simulink subsystem "untimed_ctrl"  (R2021b)
settings: Solver=VariableStepAuto  StartTime=0.0  StopTime=10.0  RelTol=1e-3
undefined symbols (not defined in the file or in its folder): ls_bitwidth
settings Model: Creator=torha  LastModifiedBy=torha
settings SolverCC: AlgebraicLoopSolver=TrustRegion
settings DebuggingCC: SFMachineParentedDataDiag=warning

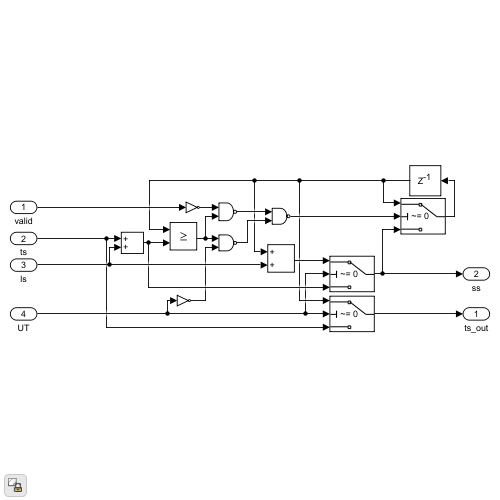
[thumbnail: Simulink's stored preview of the top-level diagram]
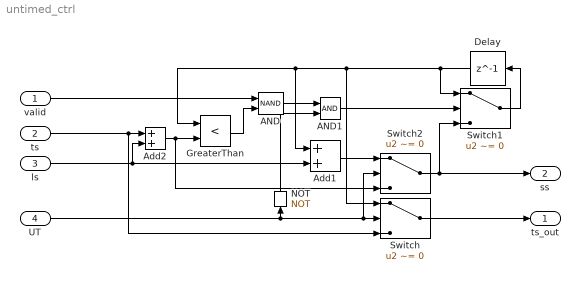
== system untimed_ctrl ==
  valid : Inport
  ts : Inport  Port=2
  ls : Inport  Port=3
  UT : Inport  Port=4
  AND : Logic  Operator=NAND  IconShape=distinctive  AllPortsSameDT=off  OutDataTypeStr=boolean
  AND1 : Logic  IconShape=distinctive  AllPortsSameDT=off  OutDataTypeStr=boolean
  Add1 : Sum  AccumDataTypeStr=fixdt(0,ls_bitwidth,0)
  Add2 : Sum  AccumDataTypeStr=fixdt(0,ls_bitwidth,0)
  Delay : Delay  DelayLength=1  InitialCondition=fi(0,0,ls_bitwidth,0)
  GreaterThan : RelationalOperator  Operator=<  OutDataTypeStr=boolean  RndMeth=Simplest
  NOT : Logic  Operator=NOT  IconShape=distinctive  AllPortsSameDT=off  OutDataTypeStr=boolean
  Switch : Switch  Criteria=u2 ~= 0
  Switch1 : Switch  Criteria=u2 ~= 0
  Switch2 : Switch  Criteria=u2 ~= 0
  ts_out : Outport
  ss : Outport  Port=2
  wires:
  ls/1 -> Add1/2, Add2/2
  Add1/1 -> Switch2/1
  Switch2/1 -> Switch1/3, ss/1
  Add2/1 -> Switch2/3, GreaterThan/2
  Delay/1 -> Switch1/1, Add1/1, GreaterThan/1, Switch/1
  Switch1/1 -> Delay/1
  UT/1 -> Switch/2, Switch2/2, NOT/1
  Switch/1 -> ts_out/1
  ts/1 -> Switch/3, Add2/1
  valid/1 -> AND/1
  GreaterThan/1 -> AND/2
  AND/1 -> AND1/1
  AND1/1 -> Switch1/2
  NOT/1 -> AND1/2
